simulink model "momentum_envelope_test_failed"  (R2018b)
settings: Solver=ode4  StartTime=0.0  StopTime=500  FixedStep=0.1  RelTol=1e-3
values from neighbouring files (symbols this model uses):
  A_failed = fswParams.allocator.rwa.A    [momentum_envelop_test_failed_init.m]
  rwa_valid = [ true; true; true; true ]    [momentum_envelop_test_failed_init.m]
undefined symbols (not defined in the file or in its folder): DiscIntNeverNeededParam, fswParams
libraries: rwa_allocation_lib x1
settings Model: Creator=taylorreynolds  LastModifiedBy=taylorreynolds

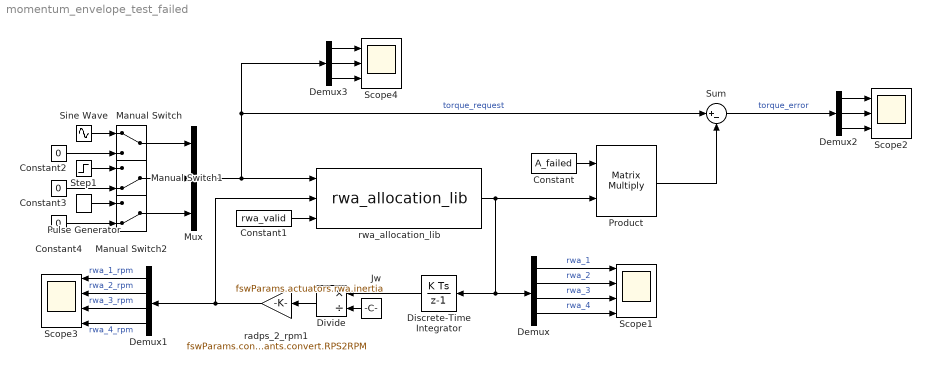
== system momentum_envelope_test_failed ==
  Constant : Constant  Value=A_failed
  Constant1 : Constant  Value=rwa_valid
  Constant2 : Constant  Value=0
  Constant3 : Constant  Value=0
  Constant4 : Constant  Value=0
  Demux : Demux
  Demux1 : Demux
  Demux2 : Demux  Outputs=3
  Demux3 : Demux  Outputs=3
  Discrete-Time Integrator : DiscreteIntegrator  SampleTime=-1  ICPrevOutput=DiscIntNeverNeededParam  ICPrevScaledInput=DiscIntNeverNeededParam
  Divide : Product  Inputs=*/
  Jw : Constant  Value=fswParams.actuators.rwa.inertia
  Manual Switch : ManualSwitch
  Manual Switch1 : ManualSwitch  CurrentSetting=0
  Manual Switch2 : ManualSwitch  CurrentSetting=0
  Mux : Mux  Inputs=3
  Product : Product  Multiplication=Matrix(*)
  Pulse Generator : DiscretePulseGenerator  PulseType=Time based  Amplitude=1e-3  Period=60  PulseWidth=5
  Scope1 : Scope  NumInputPorts=4
  Scope2 : Scope  NumInputPorts=3
  Scope3 : Scope  NumInputPorts=4
  Scope4 : Scope  NumInputPorts=3
  Sine Wave : Sin  Amplitude=1e-4  Frequency=0.1  SampleTime=0
  Step1 : Step  After=1e-4  SampleTime=0
  Sum : Sum  Inputs=|+-
  radps_2_rpm1 : Gain  Gain=fswParams.constants.convert.RPS2RPM
  rwa_allocation_lib : rwa_allocation_lib/rwa_allocation_lib  SystemSampleTime=-1
  wires:
  Demux1/1 -> Scope3/1  "rwa_1_rpm"
  radps_2_rpm1/1 -> rwa_allocation_lib/2, Demux1/1
  Demux/1 -> Scope1/1  "rwa_1"
  Discrete-Time Integrator/1 -> Divide/1
  Constant1/1 -> rwa_allocation_lib/3
  Demux/4 -> Scope1/4  "rwa_4"
  Demux1/4 -> Scope3/4  "rwa_4_rpm"
  Product/1 -> Sum/2
  Demux2/1 -> Scope2/1
  Demux/2 -> Scope1/2  "rwa_2"
  Demux/3 -> Scope1/3  "rwa_3"
  Demux1/2 -> Scope3/2  "rwa_2_rpm"
  Demux1/3 -> Scope3/3  "rwa_3_rpm"
  Demux2/2 -> Scope2/2
  Demux2/3 -> Scope2/3
  Divide/1 -> radps_2_rpm1/1
  Constant/1 -> Product/1
  rwa_allocation_lib/1 -> Product/2, Discrete-Time Integrator/1, Demux/1
  Demux3/3 -> Scope4/3
  Demux3/2 -> Scope4/2
  Demux3/1 -> Scope4/1
  Mux/1 -> rwa_allocation_lib/1, Demux3/1, Sum/1  "torque_request"
  Sum/1 -> Demux2/1  "torque_error"
  Manual Switch1/1 -> Mux/2
  Constant2/1 -> Manual Switch/2
  Sine Wave/1 -> Manual Switch/1
  Step1/1 -> Manual Switch1/1
  Constant3/1 -> Manual Switch1/2
  Manual Switch2/1 -> Mux/3
  Manual Switch/1 -> Mux/1
  Constant4/1 -> Manual Switch2/2
  Pulse Generator/1 -> Manual Switch2/1
  Jw/1 -> Divide/2
